simulink model "CLIK_Jinv"  (R2023b)
settings: Solver=ode1  StartTime=0.0  StopTime=50  FixedStep=Tc  RelTol=1e-3
values from neighbouring files (symbols this model uses):
  Tc = 0.001    [scara_parameters.m]
undefined symbols (not defined in the file or in its folder): DiscIntNeverNeededParam, K_Jinv, q0
settings Model: Creator=emman  LastModifiedBy=emman

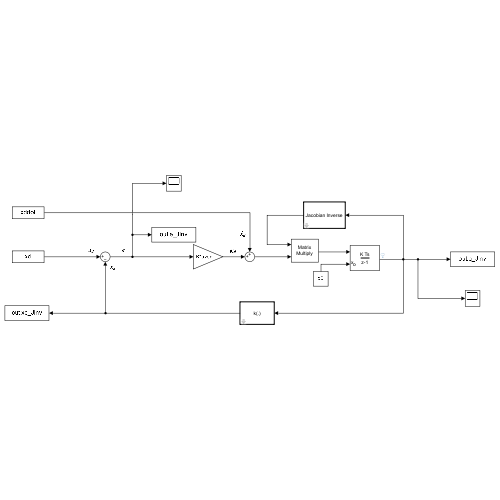
[thumbnail: Simulink's stored preview of the top-level diagram]
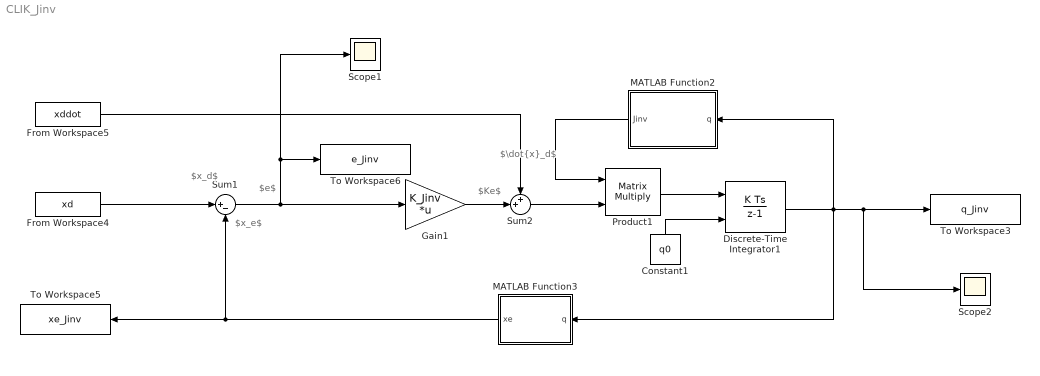
== system CLIK_Jinv ==
  note: $Ke$
  note: $e$
  note: $\dot{x}_d$
  note: $x_d$
  note: $x_e$
  Constant1 : Constant  Value=q0
  Discrete-Time Integrator1 : DiscreteIntegrator  InitialConditionSource=external  InitialCondition=q0  SampleTime=Tc  ICPrevOutput=DiscIntNeverNeededParam  ICPrevScaledInput=DiscIntNeverNeededParam
  From Workspace4 : FromWorkspace  VariableName=xd  SampleTime=Tc
  From Workspace5 : FromWorkspace  VariableName=xddot  SampleTime=Tc
  Gain1 : Gain  Gain=K_Jinv  Multiplication=Matrix(K*u) (u vector)
  MATLAB Function2 : MATLAB Function  TreatAsAtomicUnit=on
  MATLAB Function3 : MATLAB Function  TreatAsAtomicUnit=on
  Product1 : Product  Multiplication=Matrix(*)
  Scope1 : Scope
  Scope2 : Scope
  Sum1 : Sum  Inputs=|+-
  Sum2 : Sum  Inputs=++|
  To Workspace3 : ToWorkspace  VariableName=q_Jinv  SaveFormat=Structure With Time  SampleTime=-1
  To Workspace5 : ToWorkspace  VariableName=xe_Jinv  SaveFormat=Structure With Time  SampleTime=-1
  To Workspace6 : ToWorkspace  VariableName=e_Jinv  SaveFormat=Structure With Time  SampleTime=-1
  wires:
  Discrete-Time Integrator1/1 -> MATLAB Function2/1(q), To Workspace3/1, Scope2/1, MATLAB Function3/1(q)
  From Workspace4/1 -> Sum1/1
  MATLAB Function3/1(xe) -> To Workspace5/1, Sum1/2
  From Workspace5/1 -> Sum2/1
  Constant1/1 -> Discrete-Time Integrator1/2
  MATLAB Function2/1(Jinv) -> Product1/1
  Gain1/1 -> Sum2/2
  Sum2/1 -> Product1/2
  Product1/1 -> Discrete-Time Integrator1/1
  Sum1/1 -> Scope1/1, To Workspace6/1, Gain1/1

== matlab function CLIK_Jinv/MATLAB Function3 ==
  data: q input; xe output
function xe = DirKin(q)

    xe = k(q);

end

== matlab function CLIK_Jinv/MATLAB Function2 ==
  data: Jinv output; q input
function Jinv = JacobianInverse(q)

J = jacobian(q);

Jinv = inv(J);

end
